simulink model "feixianxing_4"  (R2022b)
settings: Solver=VariableStepAuto  StartTime=0.0  StopTime=10  RelTol=1e-3
settings Model: Creator=HONOR  LastModifiedBy=acer
settings DebuggingCC: UnconnectedInputMsg=warning  UnconnectedOutputMsg=warning  UnconnectedLineMsg=warning
settings ModelReferenceCC: EnableRefExpFcnMdlSchedulingChecks=on
settings RTWCC: DLArmComputeVersion=19.05

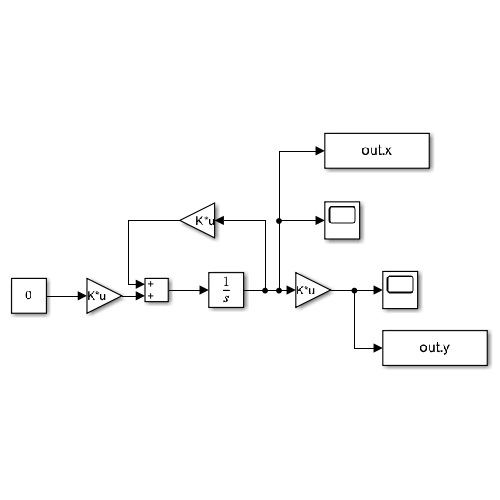
[thumbnail: Simulink's stored preview of the top-level diagram]
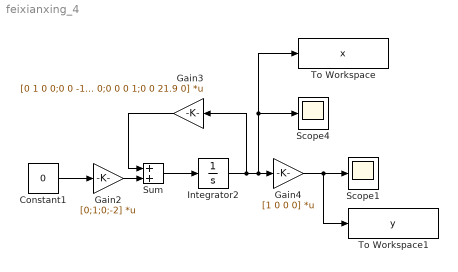
== system feixianxing_4 ==
  Constant1 : Constant  Value=0
  Gain2 : Gain  Gain=[0;1;0;-2]  Multiplication=Matrix(K*u)
  Gain3 : Gain  Gain=[0 1 0 0;0 0 -1 0;0 0 0 1;0 0 21.9 0]  Multiplication=Matrix(K*u)
  Gain4 : Gain  Gain=[1 0 0 0]  Multiplication=Matrix(K*u)
  Integrator2 : Integrator  InitialCondition=[0,0,0.1,0]
  Scope1 : Scope
  Scope4 : Scope
  Sum : Sum
  To Workspace : ToWorkspace  VariableName=x  SaveFormat=Structure With Time  SampleTime=-1
  To Workspace1 : ToWorkspace  VariableName=y  SaveFormat=Structure With Time  SampleTime=-1
  wires:
  Gain4/1 -> To Workspace1/1, Scope1/1
  Constant1/1 -> Gain2/1
  Gain3/1 -> Sum/1
  Sum/1 -> Integrator2/1
  Integrator2/1 -> Gain3/1, To Workspace/1, Scope4/1, Gain4/1
  Gain2/1 -> Sum/2
